simulink model "SpearheadSimulation"  (R2022a)
settings: Solver=ode4  StartTime=0.0  StopTime=250  RelTol=1e-3
values from neighbouring files (symbols this model uses):
  adb = importdata('datafiles/mga_v2_adb.dat')    [adbCoefficientModel.m]    (also in spearheadAnalysis.m = importdata('datafiles/adb_w_hat.txt'); spearheadControl.m = importdata('spearheadData/ConfigurationData/adb_w_hat.txt'); spearheadControl2.m = importdata('spearheadData/ConfigurationData/adb_w_hat.txt'); spearheadCruiseAnalysis.m = importdata('spearheadData/ConfigurationData/adb_w_hat.txt'))
  l_elevon = importdata('datafiles/le_w_hat.txt')    [spearheadAnalysis.m]    (also in spearheadControl.m = importdata('spearheadData/ConfigurationData/le_w_hat.txt'); spearheadControl2.m = importdata('spearheadData/ConfigurationData/le_w_hat.txt'); surfaceCoefficientModel.m = importdata('datafiles/l_elevon.dat'))
  r_elevon = importdata('datafiles/re_w_hat.txt')    [spearheadAnalysis.m]    (also in spearheadControl.m = importdata('spearheadData/ConfigurationData/re_w_hat.txt'); spearheadControl2.m = importdata('spearheadData/ConfigurationData/re_w_hat.txt'); surfaceCoefficientModel.m = importdata('datafiles/r_elevon.dat'))
  rudder = importdata('datafiles/rudder_w_hat.txt')    [spearheadAnalysis.m]    (also in spearheadControl.m = importdata('spearheadData/ConfigurationData/rudder_w_hat.txt; spearheadControl2.m = importdata('spearheadData/ConfigurationData/rudder_w_hat.txt; surfaceCoefficientModel.m = importdata('datafiles/rudder.dat'))
  T = pascal(max(dim,deg))    [makepolymat.m]    (also in spearheadAnalysis.m = 0.01; spearheadControl.m = 0.01; spearheadControl2.m = 0.01; spearheadVerticalAnalysis.m = 0.01)
libraries: slpidlib x19, simulink x5, vrlib x2, aerolibanim x1, aerolibanimutils x1
(part 2 of 2)

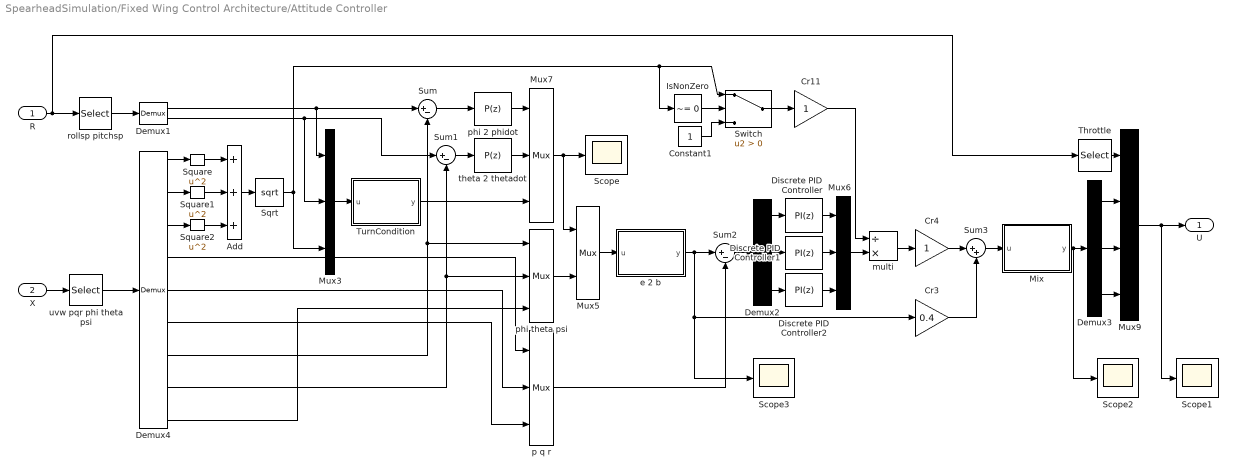
== system SpearheadSimulation/Fixed Wing Control Architecture/Attitude Controller ==
  R : Inport
  X : Inport  Port=2
  Add : Sum  Inputs=+++
  Constant1 : Constant
  Cr11 : Gain
  Cr3 : Gain  Gain=0.4
  Cr4 : Gain
  Demux1 : Demux  Outputs=2
  Demux2 : Demux  Outputs=3
  Demux3 : Demux  Outputs=3
  Demux4 : Demux  Outputs=9
  Discrete PID Controller : slpidlib/PID Controller  Controller=PI  Form=Parallel  TimeDomain=Discrete-time  UseExternalTs=off  SampleTime=-1  IntegratorMethod=Trapezoidal  FilterMethod=Trapezoidal  ControllerParametersSource=internal  P=5  I=0.5  UseKiTs=off  D=0  N=100  UseFilter=on  TunerSelectOption=Transfer Function Based (PID Tuner App)  InitialConditionSource=internal  InitialConditionForIntegrator=0  InitialConditionForFilter=0  DifferentiatorICPrevScaledInput=0  ExternalReset=none  TrackingMode=off  Kt=1  LimitOutput=off  SatLimitsSource=internal  UpperSaturationLimit=inf  LowerSaturationLimit=-inf  LinearizeAsGain=off  AntiWindupMode=none  Kb=1  POutMin=[]  POutMax=[]  IOutMin=[]  IOutMax=[]  DOutMin=[]  DOutMax=[]  NOutMin=[]  NOutMax=[]  SumOutMin=[]  SumOutMax=[]  SaturationOutMin=[]  SaturationOutMax=[]  PParamMin=[]  PParamMax=[]  IParamMin=[]  IParamMax=[]  DParamMin=[]  DParamMax=[]  NParamMin=[]  NParamMax=[]  KbParamMin=[]  KbParamMax=[]  KtParamMin=[]  KtParamMax=[]  KbOutMin=[]  KbOutMax=[]  KtOutMin=[]  KtOutMax=[]  IntegratorOutMin=[]  IntegratorOutMax=[]  FilterOutMin=[]  FilterOutMax=[]  SumI1OutMin=[]  SumI1OutMax=[]  SumI2OutMin=[]  SumI2OutMax=[]  SumI3OutMin=[]  SumI3OutMax=[]  SumI4OutMin=[]  SumI4OutMax=[]  SumDOutMin=[]  SumDOutMax=[]  DifferentiatorOutMin=[]  DifferentiatorOutMax=[]  FilterDiffOutCoefMin=[]  FilterDiffOutCoefMax=[]  ReciprocalOutMin=[]  ReciprocalOutMax=[]  SumDenOutMin=[]  SumDenOutMax=[]  SumNumOutMin=[]  SumNumOutMax=[]  DivideOutMin=[]  DivideOutMax=[]  UdiffTsProdOutMin=[]  UdiffTsProdOutMax=[]  NTsProdOutMin=[]  NTsProdOutMax=[]  UintegralTsProdOutMin=[]  UintegralTsProdOutMax=[]  UngainTsProdOutMin=[]  UngainTsProdOutMax=[]  IntegratorContinuousStateAttributes=''  IntegratorStateMustResolveToSignalObject=off  IntegratorRTWStateStorageClass=Auto  FilterContinuousStateAttributes=''  FilterStateMustResolveToSignalObject=off  FilterRTWStateStorageClass=Auto  ParallelPVariant=InternalParameters  IdealPVariant=Disabled  IVariant=InternalParameters  DVariant=Disabled  IntegratorVariant=Discrete  SatVariant=Disabled  AWVariant=Passthrough  PCopyVariant=Disabled  TRVariant=Disabled  FdbkBlocksVariant=Forward  IdealPFdbkVariant=Disabled  SatFdbkVariant=Disabled  DerivativeFilterVariant=Disabled  NVariant=Disabled  NCopyVariant=Disabled_SignalSpec  FilterICVariant=Disabled  IntegratorICVariant=InternalICs  ExternalResetVariant=Disabled  TRSumVariant=Passthrough  SumFdbkVariant=Disabled  SumVariant=Sum_PI  TsampFilterVariant=InternalTs  TsampNgainVariant=Passthrough  TsampIntegralVariant=Passthrough  ExternalSaturationOutDataTypeStr=Inherit: Same as second input  aMode=0
  Discrete PID Controller1 : slpidlib/PID Controller  Controller=PI  Form=Parallel  TimeDomain=Discrete-time  UseExternalTs=off  SampleTime=-1  IntegratorMethod=Trapezoidal  FilterMethod=Trapezoidal  ControllerParametersSource=internal  P=5  I=0.5  UseKiTs=off  D=0  N=100  UseFilter=on  TunerSelectOption=Transfer Function Based (PID Tuner App)  InitialConditionSource=internal  InitialConditionForIntegrator=0  InitialConditionForFilter=0  DifferentiatorICPrevScaledInput=0  ExternalReset=none  TrackingMode=off  Kt=1  LimitOutput=off  SatLimitsSource=internal  UpperSaturationLimit=inf  LowerSaturationLimit=-inf  LinearizeAsGain=off  AntiWindupMode=none  Kb=1  POutMin=[]  POutMax=[]  IOutMin=[]  IOutMax=[]  DOutMin=[]  DOutMax=[]  NOutMin=[]  NOutMax=[]  SumOutMin=[]  SumOutMax=[]  SaturationOutMin=[]  SaturationOutMax=[]  PParamMin=[]  PParamMax=[]  IParamMin=[]  IParamMax=[]  DParamMin=[]  DParamMax=[]  NParamMin=[]  NParamMax=[]  KbParamMin=[]  KbParamMax=[]  KtParamMin=[]  KtParamMax=[]  KbOutMin=[]  KbOutMax=[]  KtOutMin=[]  KtOutMax=[]  IntegratorOutMin=[]  IntegratorOutMax=[]  FilterOutMin=[]  FilterOutMax=[]  SumI1OutMin=[]  SumI1OutMax=[]  SumI2OutMin=[]  SumI2OutMax=[]  SumI3OutMin=[]  SumI3OutMax=[]  SumI4OutMin=[]  SumI4OutMax=[]  SumDOutMin=[]  SumDOutMax=[]  DifferentiatorOutMin=[]  DifferentiatorOutMax=[]  FilterDiffOutCoefMin=[]  FilterDiffOutCoefMax=[]  ReciprocalOutMin=[]  ReciprocalOutMax=[]  SumDenOutMin=[]  SumDenOutMax=[]  SumNumOutMin=[]  SumNumOutMax=[]  DivideOutMin=[]  DivideOutMax=[]  UdiffTsProdOutMin=[]  UdiffTsProdOutMax=[]  NTsProdOutMin=[]  NTsProdOutMax=[]  UintegralTsProdOutMin=[]  UintegralTsProdOutMax=[]  UngainTsProdOutMin=[]  UngainTsProdOutMax=[]  IntegratorContinuousStateAttributes=''  IntegratorStateMustResolveToSignalObject=off  IntegratorRTWStateStorageClass=Auto  FilterContinuousStateAttributes=''  FilterStateMustResolveToSignalObject=off  FilterRTWStateStorageClass=Auto  ParallelPVariant=InternalParameters  IdealPVariant=Disabled  IVariant=InternalParameters  DVariant=Disabled  IntegratorVariant=Discrete  SatVariant=Disabled  AWVariant=Passthrough  PCopyVariant=Disabled  TRVariant=Disabled  FdbkBlocksVariant=Forward  IdealPFdbkVariant=Disabled  SatFdbkVariant=Disabled  DerivativeFilterVariant=Disabled  NVariant=Disabled  NCopyVariant=Disabled_SignalSpec  FilterICVariant=Disabled  IntegratorICVariant=InternalICs  ExternalResetVariant=Disabled  TRSumVariant=Passthrough  SumFdbkVariant=Disabled  SumVariant=Sum_PI  TsampFilterVariant=InternalTs  TsampNgainVariant=Passthrough  TsampIntegralVariant=Passthrough  ExternalSaturationOutDataTypeStr=Inherit: Same as second input  aMode=0
  Discrete PID Controller2 : slpidlib/PID Controller  Controller=PI  Form=Parallel  TimeDomain=Discrete-time  UseExternalTs=off  SampleTime=-1  IntegratorMethod=Trapezoidal  FilterMethod=Trapezoidal  ControllerParametersSource=internal  P=5  I=0.5  UseKiTs=off  D=0  N=100  UseFilter=on  TunerSelectOption=Transfer Function Based (PID Tuner App)  InitialConditionSource=internal  InitialConditionForIntegrator=0  InitialConditionForFilter=0  DifferentiatorICPrevScaledInput=0  ExternalReset=none  TrackingMode=off  Kt=1  LimitOutput=off  SatLimitsSource=internal  UpperSaturationLimit=inf  LowerSaturationLimit=-inf  LinearizeAsGain=off  AntiWindupMode=none  Kb=1  POutMin=[]  POutMax=[]  IOutMin=[]  IOutMax=[]  DOutMin=[]  DOutMax=[]  NOutMin=[]  NOutMax=[]  SumOutMin=[]  SumOutMax=[]  SaturationOutMin=[]  SaturationOutMax=[]  PParamMin=[]  PParamMax=[]  IParamMin=[]  IParamMax=[]  DParamMin=[]  DParamMax=[]  NParamMin=[]  NParamMax=[]  KbParamMin=[]  KbParamMax=[]  KtParamMin=[]  KtParamMax=[]  KbOutMin=[]  KbOutMax=[]  KtOutMin=[]  KtOutMax=[]  IntegratorOutMin=[]  IntegratorOutMax=[]  FilterOutMin=[]  FilterOutMax=[]  SumI1OutMin=[]  SumI1OutMax=[]  SumI2OutMin=[]  SumI2OutMax=[]  SumI3OutMin=[]  SumI3OutMax=[]  SumI4OutMin=[]  SumI4OutMax=[]  SumDOutMin=[]  SumDOutMax=[]  DifferentiatorOutMin=[]  DifferentiatorOutMax=[]  FilterDiffOutCoefMin=[]  FilterDiffOutCoefMax=[]  ReciprocalOutMin=[]  ReciprocalOutMax=[]  SumDenOutMin=[]  SumDenOutMax=[]  SumNumOutMin=[]  SumNumOutMax=[]  DivideOutMin=[]  DivideOutMax=[]  UdiffTsProdOutMin=[]  UdiffTsProdOutMax=[]  NTsProdOutMin=[]  NTsProdOutMax=[]  UintegralTsProdOutMin=[]  UintegralTsProdOutMax=[]  UngainTsProdOutMin=[]  UngainTsProdOutMax=[]  IntegratorContinuousStateAttributes=''  IntegratorStateMustResolveToSignalObject=off  IntegratorRTWStateStorageClass=Auto  FilterContinuousStateAttributes=''  FilterStateMustResolveToSignalObject=off  FilterRTWStateStorageClass=Auto  ParallelPVariant=InternalParameters  IdealPVariant=Disabled  IVariant=InternalParameters  DVariant=Disabled  IntegratorVariant=Discrete  SatVariant=Disabled  AWVariant=Passthrough  PCopyVariant=Disabled  TRVariant=Disabled  FdbkBlocksVariant=Forward  IdealPFdbkVariant=Disabled  SatFdbkVariant=Disabled  DerivativeFilterVariant=Disabled  NVariant=Disabled  NCopyVariant=Disabled_SignalSpec  FilterICVariant=Disabled  IntegratorICVariant=InternalICs  ExternalResetVariant=Disabled  TRSumVariant=Passthrough  SumFdbkVariant=Disabled  SumVariant=Sum_PI  TsampFilterVariant=InternalTs  TsampNgainVariant=Passthrough  TsampIntegralVariant=Passthrough  ExternalSaturationOutDataTypeStr=Inherit: Same as second input  aMode=0
  IsNonZero : simulink/Logic and Bit Operations/Compare To Zero  relop=~=  OutDataTypeStr=boolean
  Mix : MATLAB Function  TreatAsAtomicUnit=on  SystemSampleTime=T
  Mux3 : Mux  Inputs=3
  Mux5 : Mux  Inputs=2
  Mux6 : Mux  Inputs=3
  Mux7 : Mux  Inputs=3
  Mux9 : Mux
  Scope{,1..3} (4 alike) : Scope
  Sqrt : Sqrt  OutputSignalType=real
  Square : Math  Operator=square
  Square1 : Math  Operator=square
  Square2 : Math  Operator=square
  Sum : Sum  Inputs=|+-
  Sum1 : Sum  Inputs=|+-
  Sum2 : Sum  Inputs=|+-
  Sum3 : Sum  Inputs=|++
  Switch : Switch  Criteria=u2 > Threshold  SaturateOnIntegerOverflow=off  InputSameDT=off
  Throttle : Selector  InputPortWidth=4  IndexOptions=Index vector (dialog)  Indices=[4]  OutputSizes=1
  TurnCondition : MATLAB Function  TreatAsAtomicUnit=on  SystemSampleTime=T
  e 2 b : MATLAB Function  TreatAsAtomicUnit=on  SystemSampleTime=T
  multi : Product  Inputs=/*
  p q r : Mux  Inputs=3
  phi 2 phidot : slpidlib/PID Controller  Controller=P  Form=Parallel  TimeDomain=Discrete-time  UseExternalTs=off  SampleTime=-1  IntegratorMethod=Trapezoidal  FilterMethod=Trapezoidal  ControllerParametersSource=internal  P=100  I=1  UseKiTs=off  D=0  N=100  UseFilter=on  TunerSelectOption=Transfer Function Based (PID Tuner App)  InitialConditionSource=internal  InitialConditionForIntegrator=0  InitialConditionForFilter=0  DifferentiatorICPrevScaledInput=0  ExternalReset=none  TrackingMode=off  Kt=1  LimitOutput=off  SatLimitsSource=internal  UpperSaturationLimit=inf  LowerSaturationLimit=-inf  LinearizeAsGain=off  AntiWindupMode=none  Kb=1  POutMin=[]  POutMax=[]  IOutMin=[]  IOutMax=[]  DOutMin=[]  DOutMax=[]  NOutMin=[]  NOutMax=[]  SumOutMin=[]  SumOutMax=[]  SaturationOutMin=[]  SaturationOutMax=[]  PParamMin=[]  PParamMax=[]  IParamMin=[]  IParamMax=[]  DParamMin=[]  DParamMax=[]  NParamMin=[]  NParamMax=[]  KbParamMin=[]  KbParamMax=[]  KtParamMin=[]  KtParamMax=[]  KbOutMin=[]  KbOutMax=[]  KtOutMin=[]  KtOutMax=[]  IntegratorOutMin=[]  IntegratorOutMax=[]  FilterOutMin=[]  FilterOutMax=[]  SumI1OutMin=[]  SumI1OutMax=[]  SumI2OutMin=[]  SumI2OutMax=[]  SumI3OutMin=[]  SumI3OutMax=[]  SumI4OutMin=[]  SumI4OutMax=[]  SumDOutMin=[]  SumDOutMax=[]  DifferentiatorOutMin=[]  DifferentiatorOutMax=[]  FilterDiffOutCoefMin=[]  FilterDiffOutCoefMax=[]  ReciprocalOutMin=[]  ReciprocalOutMax=[]  SumDenOutMin=[]  SumDenOutMax=[]  SumNumOutMin=[]  SumNumOutMax=[]  DivideOutMin=[]  DivideOutMax=[]  UdiffTsProdOutMin=[]  UdiffTsProdOutMax=[]  NTsProdOutMin=[]  NTsProdOutMax=[]  UintegralTsProdOutMin=[]  UintegralTsProdOutMax=[]  UngainTsProdOutMin=[]  UngainTsProdOutMax=[]  IntegratorContinuousStateAttributes=''  IntegratorStateMustResolveToSignalObject=off  IntegratorRTWStateStorageClass=Auto  FilterContinuousStateAttributes=''  FilterStateMustResolveToSignalObject=off  FilterRTWStateStorageClass=Auto  ParallelPVariant=InternalParameters  IdealPVariant=Disabled  IVariant=Disabled  DVariant=Disabled  IntegratorVariant=Disabled  SatVariant=Disabled  AWVariant=Disabled  PCopyVariant=Disabled  TRVariant=Disabled  FdbkBlocksVariant=Forward  IdealPFdbkVariant=Disabled  SatFdbkVariant=Disabled  DerivativeFilterVariant=Disabled  NVariant=Disabled  NCopyVariant=Disabled_SignalSpec  FilterICVariant=Disabled  IntegratorICVariant=Disabled  ExternalResetVariant=Disabled  TRSumVariant=Passthrough  SumFdbkVariant=Disabled  SumVariant=Passthrough_P  TsampFilterVariant=InternalTs  TsampNgainVariant=Passthrough  TsampIntegralVariant=Disabled_SignalSpec  ExternalSaturationOutDataTypeStr=Inherit: Same as second input  aMode=0
  phi theta psi : Mux  Inputs=3
  rollsp pitchsp : Selector  InputPortWidth=4  IndexOptions=Index vector (dialog)  Indices=[1,3]  OutputSizes=1
  theta 2 thetadot : slpidlib/PID Controller  Controller=P  Form=Parallel  TimeDomain=Discrete-time  UseExternalTs=off  SampleTime=-1  IntegratorMethod=Trapezoidal  FilterMethod=Trapezoidal  ControllerParametersSource=internal  P=100  I=1  UseKiTs=off  D=0  N=100  UseFilter=on  TunerSelectOption=Transfer Function Based (PID Tuner App)  InitialConditionSource=internal  InitialConditionForIntegrator=0  InitialConditionForFilter=0  DifferentiatorICPrevScaledInput=0  ExternalReset=none  TrackingMode=off  Kt=1  LimitOutput=off  SatLimitsSource=internal  UpperSaturationLimit=inf  LowerSaturationLimit=-inf  LinearizeAsGain=off  AntiWindupMode=none  Kb=1  POutMin=[]  POutMax=[]  IOutMin=[]  IOutMax=[]  DOutMin=[]  DOutMax=[]  NOutMin=[]  NOutMax=[]  SumOutMin=[]  SumOutMax=[]  SaturationOutMin=[]  SaturationOutMax=[]  PParamMin=[]  PParamMax=[]  IParamMin=[]  IParamMax=[]  DParamMin=[]  DParamMax=[]  NParamMin=[]  NParamMax=[]  KbParamMin=[]  KbParamMax=[]  KtParamMin=[]  KtParamMax=[]  KbOutMin=[]  KbOutMax=[]  KtOutMin=[]  KtOutMax=[]  IntegratorOutMin=[]  IntegratorOutMax=[]  FilterOutMin=[]  FilterOutMax=[]  SumI1OutMin=[]  SumI1OutMax=[]  SumI2OutMin=[]  SumI2OutMax=[]  SumI3OutMin=[]  SumI3OutMax=[]  SumI4OutMin=[]  SumI4OutMax=[]  SumDOutMin=[]  SumDOutMax=[]  DifferentiatorOutMin=[]  DifferentiatorOutMax=[]  FilterDiffOutCoefMin=[]  FilterDiffOutCoefMax=[]  ReciprocalOutMin=[]  ReciprocalOutMax=[]  SumDenOutMin=[]  SumDenOutMax=[]  SumNumOutMin=[]  SumNumOutMax=[]  DivideOutMin=[]  DivideOutMax=[]  UdiffTsProdOutMin=[]  UdiffTsProdOutMax=[]  NTsProdOutMin=[]  NTsProdOutMax=[]  UintegralTsProdOutMin=[]  UintegralTsProdOutMax=[]  UngainTsProdOutMin=[]  UngainTsProdOutMax=[]  IntegratorContinuousStateAttributes=''  IntegratorStateMustResolveToSignalObject=off  IntegratorRTWStateStorageClass=Auto  FilterContinuousStateAttributes=''  FilterStateMustResolveToSignalObject=off  FilterRTWStateStorageClass=Auto  ParallelPVariant=InternalParameters  IdealPVariant=Disabled  IVariant=Disabled  DVariant=Disabled  IntegratorVariant=Disabled  SatVariant=Disabled  AWVariant=Disabled  PCopyVariant=Disabled  TRVariant=Disabled  FdbkBlocksVariant=Forward  IdealPFdbkVariant=Disabled  SatFdbkVariant=Disabled  DerivativeFilterVariant=Disabled  NVariant=Disabled  NCopyVariant=Disabled_SignalSpec  FilterICVariant=Disabled  IntegratorICVariant=Disabled  ExternalResetVariant=Disabled  TRSumVariant=Passthrough  SumFdbkVariant=Disabled  SumVariant=Passthrough_P  TsampFilterVariant=InternalTs  TsampNgainVariant=Passthrough  TsampIntegralVariant=Disabled_SignalSpec  ExternalSaturationOutDataTypeStr=Inherit: Same as second input  aMode=0
  uvw pqr phi theta psi : Selector  InputPortWidth=20  IndexOptions=Index vector (dialog)  Indices=[1,2,3,4,5,6,10,11,12]  OutputSizes=1
  U : Outport
  wires:
  X/1 -> uvw pqr phi theta psi/1
  Sum1/1 -> theta 2 thetadot/1
  Sqrt/1 -> IsNonZero/1, Switch/1, Mux3/3
  Demux4/8 -> Sum1/2, phi theta psi/2
  Demux1/2 -> Sum1/1, Mux3/2
  Cr3/1 -> Sum3/2
  Mux7/1 -> Mux5/1, Scope/1
  Mux5/1 -> e 2 b/1(u)
  Cr4/1 -> Sum3/1
  rollsp pitchsp/1 -> Demux1/1
  R/1 -> rollsp pitchsp/1, Throttle/1
  Sum/1 -> phi 2 phidot/1
  Throttle/1 -> Mux9/1
  Demux4/5 -> p q r/2
  TurnCondition/1(y) -> Mux7/3
  multi/1 -> Cr4/1
  e 2 b/1(y) -> Sum2/1, Scope3/1, Cr3/1
  Demux3/1 -> Mux9/2
  phi theta psi/1 -> Mux5/2
  Mux9/1 -> Scope1/1, U/1
  Demux3/2 -> Mux9/3
  Demux4/2 -> Square1/1
  Demux1/1 -> Sum/1, Mux3/1
  Demux4/7 -> phi theta psi/1, Sum/2
  Mix/1(y) -> Scope2/1, Demux3/1
  phi 2 phidot/1 -> Mux7/1
  Mux3/1 -> TurnCondition/1(u)
  Square1/1 -> Add/2
  Sum2/1 -> Demux2/1
  Demux4/3 -> Square2/1
  Square/1 -> Add/1
  Square2/1 -> Add/3
  Add/1 -> Sqrt/1
  Demux4/4 -> p q r/1
  Sum3/1 -> Mix/1(u)
  Demux4/9 -> phi theta psi/3
  IsNonZero/1 -> Switch/2
  Demux3/3 -> Mux9/4
  Demux2/1 -> Discrete PID Controller/1
  Discrete PID Controller/1 -> Mux6/1
  Discrete PID Controller2/1 -> Mux6/3
  p q r/1 -> Sum2/2
  Switch/1 -> Cr11/1
  Demux2/3 -> Discrete PID Controller2/1
  Discrete PID Controller1/1 -> Mux6/2
  Mux6/1 -> multi/2
  Demux2/2 -> Discrete PID Controller1/1
  uvw pqr phi theta psi/1 -> Demux4/1
  Demux4/6 -> p q r/3
  Cr11/1 -> multi/1
  Demux4/1 -> Square/1
  Constant1/1 -> Switch/3
  theta 2 thetadot/1 -> Mux7/2

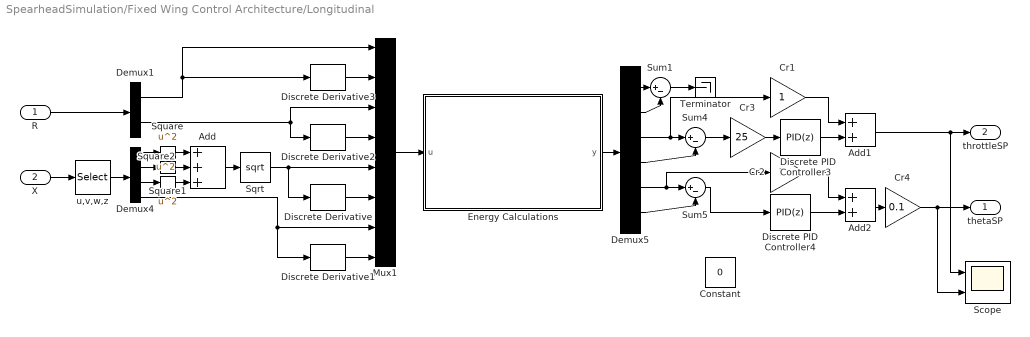
== system SpearheadSimulation/Fixed Wing Control Architecture/Longitudinal ==
  R : Inport
  X : Inport  Port=2
  Add : Sum  Inputs=+++
  Add1 : Sum
  Add2 : Sum
  Constant : Constant  Value=0
  Cr1 : Gain
  Cr2 : Gain
  Cr3 : Gain  Gain=25
  Cr4 : Gain  Gain=0.1
  Demux1 : Demux  Outputs=2
  Demux4 : Demux
  Demux5 : Demux  Outputs=6
  Discrete Derivative{,1..3} (4 alike) : simulink/Discrete/Discrete Derivative  gainval=1.0  ICPrevScaledInput=0.0  OutMin=[]  OutMax=[]  OutDataType=fixdt(1, 16)  OutScaling=2^-10  DoSatur=off
  Discrete PID Controller3 : slpidlib/PID Controller  Controller=PID  Form=Parallel  TimeDomain=Discrete-time  UseExternalTs=off  SampleTime=-1  IntegratorMethod=Trapezoidal  FilterMethod=Trapezoidal  ControllerParametersSource=internal  P=1  I=1/5  UseKiTs=off  D=1/25  N=100  UseFilter=on  TunerSelectOption=Transfer Function Based (PID Tuner App)  InitialConditionSource=internal  InitialConditionForIntegrator=0  InitialConditionForFilter=0  DifferentiatorICPrevScaledInput=0  ExternalReset=none  TrackingMode=off  Kt=1  LimitOutput=off  SatLimitsSource=internal  UpperSaturationLimit=inf  LowerSaturationLimit=-inf  LinearizeAsGain=off  AntiWindupMode=none  Kb=1  POutMin=[]  POutMax=[]  IOutMin=[]  IOutMax=[]  DOutMin=[]  DOutMax=[]  NOutMin=[]  NOutMax=[]  SumOutMin=[]  SumOutMax=[]  SaturationOutMin=[]  SaturationOutMax=[]  PParamMin=[]  PParamMax=[]  IParamMin=[]  IParamMax=[]  DParamMin=[]  DParamMax=[]  NParamMin=[]  NParamMax=[]  KbParamMin=[]  KbParamMax=[]  KtParamMin=[]  KtParamMax=[]  KbOutMin=[]  KbOutMax=[]  KtOutMin=[]  KtOutMax=[]  IntegratorOutMin=[]  IntegratorOutMax=[]  FilterOutMin=[]  FilterOutMax=[]  SumI1OutMin=[]  SumI1OutMax=[]  SumI2OutMin=[]  SumI2OutMax=[]  SumI3OutMin=[]  SumI3OutMax=[]  SumI4OutMin=[]  SumI4OutMax=[]  SumDOutMin=[]  SumDOutMax=[]  DifferentiatorOutMin=[]  DifferentiatorOutMax=[]  FilterDiffOutCoefMin=[]  FilterDiffOutCoefMax=[]  ReciprocalOutMin=[]  ReciprocalOutMax=[]  SumDenOutMin=[]  SumDenOutMax=[]  SumNumOutMin=[]  SumNumOutMax=[]  DivideOutMin=[]  DivideOutMax=[]  UdiffTsProdOutMin=[]  UdiffTsProdOutMax=[]  NTsProdOutMin=[]  NTsProdOutMax=[]  UintegralTsProdOutMin=[]  UintegralTsProdOutMax=[]  UngainTsProdOutMin=[]  UngainTsProdOutMax=[]  IntegratorContinuousStateAttributes=''  IntegratorStateMustResolveToSignalObject=off  IntegratorRTWStateStorageClass=Auto  FilterContinuousStateAttributes=''  FilterStateMustResolveToSignalObject=off  FilterRTWStateStorageClass=Auto  ParallelPVariant=InternalParameters  IdealPVariant=Disabled  IVariant=InternalParameters  DVariant=InternalParameters  IntegratorVariant=Discrete  SatVariant=Disabled  AWVariant=Passthrough  PCopyVariant=Disabled  TRVariant=Disabled  FdbkBlocksVariant=Forward  IdealPFdbkVariant=Disabled  SatFdbkVariant=Disabled  DerivativeFilterVariant=TrapezoidalFilter  NVariant=InternalParameters  NCopyVariant=InternalParameters  FilterICVariant=InternalICsFilter  IntegratorICVariant=InternalICs  ExternalResetVariant=Disabled  TRSumVariant=Passthrough  SumFdbkVariant=Disabled  SumVariant=Sum_PID  TsampFilterVariant=InternalTs  TsampNgainVariant=Passthrough  TsampIntegralVariant=Passthrough  ExternalSaturationOutDataTypeStr=Inherit: Same as second input  aMode=0
  Discrete PID Controller4 : slpidlib/PID Controller  Controller=PID  Form=Parallel  TimeDomain=Discrete-time  UseExternalTs=off  SampleTime=-1  IntegratorMethod=Trapezoidal  FilterMethod=Trapezoidal  ControllerParametersSource=internal  P=20  I=1  UseKiTs=off  D=10  N=100  UseFilter=on  TunerSelectOption=Transfer Function Based (PID Tuner App)  InitialConditionSource=internal  InitialConditionForIntegrator=0  InitialConditionForFilter=0  DifferentiatorICPrevScaledInput=0  ExternalReset=none  TrackingMode=off  Kt=1  LimitOutput=off  SatLimitsSource=internal  UpperSaturationLimit=inf  LowerSaturationLimit=-inf  LinearizeAsGain=off  AntiWindupMode=none  Kb=1  POutMin=[]  POutMax=[]  IOutMin=[]  IOutMax=[]  DOutMin=[]  DOutMax=[]  NOutMin=[]  NOutMax=[]  SumOutMin=[]  SumOutMax=[]  SaturationOutMin=[]  SaturationOutMax=[]  PParamMin=[]  PParamMax=[]  IParamMin=[]  IParamMax=[]  DParamMin=[]  DParamMax=[]  NParamMin=[]  NParamMax=[]  KbParamMin=[]  KbParamMax=[]  KtParamMin=[]  KtParamMax=[]  KbOutMin=[]  KbOutMax=[]  KtOutMin=[]  KtOutMax=[]  IntegratorOutMin=[]  IntegratorOutMax=[]  FilterOutMin=[]  FilterOutMax=[]  SumI1OutMin=[]  SumI1OutMax=[]  SumI2OutMin=[]  SumI2OutMax=[]  SumI3OutMin=[]  SumI3OutMax=[]  SumI4OutMin=[]  SumI4OutMax=[]  SumDOutMin=[]  SumDOutMax=[]  DifferentiatorOutMin=[]  DifferentiatorOutMax=[]  FilterDiffOutCoefMin=[]  FilterDiffOutCoefMax=[]  ReciprocalOutMin=[]  ReciprocalOutMax=[]  SumDenOutMin=[]  SumDenOutMax=[]  SumNumOutMin=[]  SumNumOutMax=[]  DivideOutMin=[]  DivideOutMax=[]  UdiffTsProdOutMin=[]  UdiffTsProdOutMax=[]  NTsProdOutMin=[]  NTsProdOutMax=[]  UintegralTsProdOutMin=[]  UintegralTsProdOutMax=[]  UngainTsProdOutMin=[]  UngainTsProdOutMax=[]  IntegratorContinuousStateAttributes=''  IntegratorStateMustResolveToSignalObject=off  IntegratorRTWStateStorageClass=Auto  FilterContinuousStateAttributes=''  FilterStateMustResolveToSignalObject=off  FilterRTWStateStorageClass=Auto  ParallelPVariant=InternalParameters  IdealPVariant=Disabled  IVariant=InternalParameters  DVariant=InternalParameters  IntegratorVariant=Discrete  SatVariant=Disabled  AWVariant=Passthrough  PCopyVariant=Disabled  TRVariant=Disabled  FdbkBlocksVariant=Forward  IdealPFdbkVariant=Disabled  SatFdbkVariant=Disabled  DerivativeFilterVariant=TrapezoidalFilter  NVariant=InternalParameters  NCopyVariant=InternalParameters  FilterICVariant=InternalICsFilter  IntegratorICVariant=InternalICs  ExternalResetVariant=Disabled  TRSumVariant=Passthrough  SumFdbkVariant=Disabled  SumVariant=Sum_PID  TsampFilterVariant=InternalTs  TsampNgainVariant=Passthrough  TsampIntegralVariant=Passthrough  ExternalSaturationOutDataTypeStr=Inherit: Same as second input  aMode=0
  Energy Calculations : MATLAB Function  TreatAsAtomicUnit=on  SystemSampleTime=T
  Mux1 : Mux  Inputs=8
  Scope : Scope  NumInputPorts=2
  Sqrt : Sqrt  OutputSignalType=real
  Square : Math  Operator=square
  Square1 : Math  Operator=square
  Square2 : Math  Operator=square
  Sum1 : Sum  Inputs=|+-
  Sum4 : Sum  Inputs=|+-
  Sum5 : Sum  Inputs=|+-
  Terminator : Terminator
  u,v,w,z : Selector  InputPortWidth=20  IndexOptions=Index vector (dialog)  Indices=[1,2,3,9]  OutputSizes=1
  thetaSP : Outport
  throttleSP : Outport  Port=2
  wires:
  X/1 -> u,v,w,z/1
  Demux4/2 -> Square1/1
  Square1/1 -> Add/2
  Demux4/3 -> Square2/1
  Square/1 -> Add/1
  Square2/1 -> Add/3
  Add/1 -> Sqrt/1
  u,v,w,z/1 -> Demux4/1
  Demux4/1 -> Square/1
  Mux1/1 -> Energy Calculations/1(u)
  Sqrt/1 -> Mux1/5, Discrete Derivative/1
  Demux4/4 -> Mux1/7, Discrete Derivative1/1
  R/1 -> Demux1/1
  Discrete Derivative1/1 -> Mux1/8
  Discrete Derivative/1 -> Mux1/6
  Demux1/2 -> Discrete Derivative2/1, Mux1/3
  Discrete Derivative2/1 -> Mux1/4
  Demux1/1 -> Discrete Derivative3/1, Mux1/1
  Discrete Derivative3/1 -> Mux1/2
  Energy Calculations/1(y) -> Demux5/1
  Demux5/1 -> Sum1/1
  Demux5/2 -> Sum1/2
  Demux5/3 -> Cr1/1, Sum4/1
  Demux5/4 -> Sum4/2
  Demux5/5 -> Cr2/1, Sum5/1
  Demux5/6 -> Sum5/2
  Discrete PID Controller3/1 -> Add1/2
  Cr1/1 -> Add1/1
  Add1/1 -> Scope/1, throttleSP/1
  Cr2/1 -> Add2/1
  Discrete PID Controller4/1 -> Add2/2
  Sum5/1 -> Discrete PID Controller4/1
  Cr3/1 -> Discrete PID Controller3/1
  Sum4/1 -> Cr3/1
  Sum1/1 -> Terminator/1
  Add2/1 -> Cr4/1
  Cr4/1 -> thetaSP/1, Scope/2

== matlab function SpearheadSimulation/SpearheadModel ==
  data: k input; dX output; X input; U input; adb input; l_elevon input; r_elevon input; rudder input
function dX  = spearheadModel(k,X,U,adb,l_elevon,r_elevon,rudder)
%% Xdot = f(X,U)

%% Mass of the VTOL Craft as Taken From CAD
M = 20;
g = 9.81;
rho = 1.225; % sea level air density

%% VTOL Dimensions
% CG at [0.6, 0, 0] m.
L1 = 1.65;
L2 = 1.425;
C = 0.32; % Wing Mean Cord Length
S = 2.24; % Wing Planform Area
eS = 0.28*0.58;% Elevon Planform Area chord x span
rS = 0.32*0.30;% Rudder Planform Area chord x span

%% Mass Moment of Inertia about the COM As Taken From CAD
Ixx = 5.061E+05;
Iyy = 5.061E+05;
Izz = 10.011E+05;

%% X = [u v w p q r x y z phi theta psi w1 w2 w3 w4 w5 dl dr drd]
% Linear and Angular Velocity in Fb (m/s and rads/s)
u = X(1);
v = X(2);
w = X(3);
p = X(4);
q = X(5);
r = X(6);
% Linear and Angular position in Fe (meters and rads)
x = X(7);
y = X(8);
z = X(9);
phi = X(10);
theta = X(11);
psi = X(12);
% Motor angular velocity (RPM)
w1 = X(13);
w2 = X(14);
w3 = X(15);
w4 = X(16);
w5 = X(17);
% Control Surface Defelection Angles(degrees)
dl = X(18);
dr = X(19);
drd = X(20);

%% U = [u1 u2 u3 u4 u5 u6 u7 u8] K = Motor Gain Mau = Time Constant Ku = Input Gain
K = [1.123*10^-6; 2.25*10^-6; 7.708*10^-7; 18.708*10^-7];
Mtau = [1/44.22; 1/44.22; 1/20];
Ku = [44.2205*8.18; 44.2205*7.02; 3.6];

F1 = K(1)*w1*w1;
F2 = K(1)*w2*w2;    
F3 = K(1)*w3*w3;
F4 = K(1)*w4*w4;

F5 = K(2)*w5*w5;

Tau1 = K(3)*w1*w1;
Tau2 = -K(3)*w2*w2;
Tau3 = -K(3)*w3*w3;
Tau4 = K(3)*w4*w4;

Tau5 = K(4)*w5*w5;

Fn = F1+F2+F3+F4;
Taun = Tau1+Tau2+Tau3+Tau4;

%% Wind Frame Variables: V = Airspeed alpha = AngleofAttack beta = AngleofSideslip
todeg = 180/pi;
V = sqrt(u*u + v*v + w*w);
alpha = atan2(w,u)*todeg;

if V == 0
  beta = 0;
else
  beta = asin(v/V)*todeg;
end

%% Aerodynamic Coefficients: ['CFX','CFY','CFZ','CMX','CMY','CMZ']
adb_C = adbCoefficients(alpha,beta,adb);
le_C = [1 dl dl^2 dl^3 dl^4 dl^5 dl^6 dl^7 dl^8]*l_elevon;
re_C = [1 dr dr^2 dr^3 dr^4 dr^5 dr^6 dr^7 dr^8]*r_elevon;
rudder_C = [1 drd drd^2 drd^3 drd^4 drd^5 drd^6 drd^7 drd^8]*rudder;

%% Forces: Thrust
FTx = F5;
FTy = 0;
FTz = -Fn;

%% Forces: Gravity
FGx = -g*sin(theta);
FGy = g*sin(phi)*cos(theta);
FGz = g*cos(phi)*cos(theta);

%% Forces: Aerodynamic [Drag,Sideforce,Lift]
FAx = 0.5 * rho * V*V * (S * adb_C(1) + eS * le_C(1) + eS * re_C(1) + rS * rudder_C(1));
FAy = 0.5 * rho * V*V * (S * adb_C(2) + eS * le_C(2) + eS * re_C(2) + rS * rudder_C(2));
FAz = 0.5 * rho * V*V * (S * adb_C(3) + eS * le_C(3) + eS * re_C(3) + rS * rudder_C(3));

%% Moments: Thrust
LT = L1*((F1 + F3) - (F2 + F4)) + Tau5;
MT = L2*((F1 + F2) - (F3 + F4));
NT = Taun;

%% Moments: Aerodynamic [Roll,Pitch,Yaw]
LA = 0.5 * rho * V*V * C * (S * adb_C(4) + eS * le_C(4) + eS * re_C(4) + rS * rudder_C(4));
MA = 0.5 * rho * V*V * C * (S * adb_C(5) + eS * le_C(5) + eS * re_C(5) + rS * rudder_C(5));
NA = 0.5 * rho * V*V * C * (S * adb_C(6) + eS * le_C(6) + eS * re_C(6) + rS * rudder_C(6));

%% 6-DOF Dynamics: dX = [udot vdot wdot pdot qdot rdot xdot ydot zdot phidot thetadot psidot]
dX1 = FGx + FAx/M + FTx/M - q*w + r*v;%# + g*sin(theta);
dX2 = FGy + FAy/M + FTy/M - r*u + p*w;
dX3 = FGz + FAz/M + FTz/M - p*v + q*u;%# - g*cos(theta);
dX4 = LA/Ixx + LT/Ixx - q*r*(Izz - Iyy)/Ixx;
dX5 = MA/Iyy + MT/Iyy - p*r*(Ixx - Izz)/Iyy;
dX6 = NA/Izz + NT/Izz - p*q*(Iyy - Ixx)/Izz;

dX7 = u*(cos(theta)*cos(psi)) + v*(sin(phi)*sin(theta)*cos(psi) - cos(phi)*sin(psi)) + w*(cos(phi)*sin(theta)*cos(psi) + sin(phi)*sin(psi));
dX8 = u*(cos(theta)*sin(psi)) + v*(sin(phi)*sin(theta)*sin(psi) + cos(phi)*cos(psi)) + w*(cos(phi)*sin(theta)*sin(psi) - sin(phi)*cos(psi));
dX9 = -u*(sin(theta)) + v*(sin(phi)*cos(theta)) + w*(cos(phi)*cos(theta));
dX10 = p + q*(sin(phi)*tan(theta)) + r*(cos(phi)*tan(theta));
dX11 = q*cos(phi) - r*sin(phi);
dX12 = q*(sin(phi)/cos(theta)) + r*(cos(phi)/cos(theta));

%% Motor Dynamics: dX = [w1dot w2dot w3dot w4dot w5dot], U = Pulse Width of the pwm signal 0-1000
dX13 = -(1/Mtau(1))*w1 + Ku(1)*U(1);
dX14 = -(1/Mtau(1))*w2 + Ku(1)*U(2);
dX15 = -(1/Mtau(1))*w3 + Ku(1)*U(3);
dX16 = -(1/Mtau(1))*w4 + Ku(1)*U(4);
dX17 = -(1/Mtau(2))*w5 + Ku(2)*U(5);

%% Servo Dynamics: dX = [w6dot w7dot w8dot], U = Pulse Width of the pwm signal 0-1000
dX18 = -(1/Mtau(3))*dl + Ku(3)*U(6);
dX19 = -(1/Mtau(3))*dr + Ku(3)*U(7);
dX20 = -(1/Mtau(3))*drd + Ku(3)*U(8);

dX = [dX1;dX2;dX3;dX4;dX5;dX6;dX7;dX8;dX9;dX10;dX11;dX12;dX13;dX14;dX15;dX16;dX17;dX18;dX19;dX20];
end

== matlab function SpearheadSimulation/Fixed Wing Control Architecture/Attitude Controller/e 2 b ==
  data: u input; y output
function y = etb(u)
y = [1,sin(u(4))*tan(u(5)),cos(u(4))*tan(u(5));
     0,            cos(u(4)),           -sin(u(4));
     0,sin(u(4))/cos(u(5)),cos(u(4))/cos(u(5))]\u([1,2,3]);

== matlab function SpearheadSimulation/Fixed Wing Control Architecture/Attitude Controller/TurnCondition ==
  data: u input; y output
function y = TurnCondition(u)

if u(3) == 0
    y = 0;
else
    y = (9.81/u(3)) * tan(u(1)) * cos(u(2));
end

== matlab function SpearheadSimulation/Fixed Wing Control Architecture/Attitude Controller/Mix ==
  data: u input; y output
function y = Mix(u)
y = [0.5,0.5,0;
     -0.5,0.5,0;
     0,0,1]*u;

== matlab function SpearheadSimulation/Fixed Wing Control Architecture/Longitudinal/Energy Calculations ==
  data: u input; y output
function y = Energy(u)
M = 20;
g = 9.81;

hsp = u(3);
hdotsp = u(4);
h = u(7);
hdot = u(8);
Vsp = u(1);
Vdot = u(2);
V = u(5);
Vdotsp = u(6);

Et = 0.5 * M * V^2 + M * g * h;
Etdot = M * V * Vdot + M * g * hdot;
if V == 0 
    Edot = 0;
    gamma  = 0;
else
    Edot = Etdot/(M * g * V);
    gamma = asin(abs(hdot/V));
end
Bdot = gamma - Vdot/g;

Etsp = 0.5 * M * Vsp^2 + M * g * hsp;
Etdotsp = M * Vsp * Vdotsp + M * g * hdotsp;
if Vsp == 0
    Edotsp = 0;
    gammasp  = 0;
else
    Edotsp = Etdotsp/(M * g * V);
    gammasp = asin(abs(hdotsp/Vsp));
end        
Bdotsp = gammasp - Vdotsp/g;

y = [Etsp,Et,Edotsp,Edot,Bdotsp,Bdot];
end

== matlab function SpearheadSimulation/Rotor Wing Control Architecture/Acceleration to Attitiude ==
  data: u input; y output
function y = ata(u)

collcmd =  sqrt((u(1)^2)*(u(2)^2)*(u(3)^2));

if collcmd == 0
    I = [0;0;0];
else
    I = u([1;2;3])/collcmd;
end

K = [cos(u(4)),sin(u(4)),0;
     -sin(u(4)),cos(u(4)),0;
     0,         0,       1]*I;

if collcmd == 0
    thetacmd = 0;
else
    thetacmd = atan(K(1)/K(3));
end

L = [cos(thetacmd),0,-sin(thetacmd);
        0,         1,       0;
     sin(thetacmd),0,cos(thetacmd)]*K;

if collcmd == 0
    phicmd = 0;
else
    phicmd = atan2(-L(2),L(3));
end

y = [phicmd,thetacmd,u(4),u(3)];

end

== matlab function SpearheadSimulation/Rotor Wing Control Architecture/Mix1 ==
  data: u input; y output
function y = Mix(u)
M = 20;
L1 = 1.65;
L2 = 1.425;
Ixx = 5.061E+05;
Iyy = 5.061E+05;
Izz = 10.011E+05;
K = 1.123*10^-6;
K2 = 7.708*10^-7;
Ku = 44.2205*8.18;

%{
Usqr = [L1*K/Ixx, -L1*K/Ixx, L1*K/Ixx, -L1*K/Ixx;
        L2*K/Iyy, L2*K/Iyy, -L2*K/Iyy, -L2*K/Iyy;
        K2/Izz,    -K2/Izz,   -K2/Izz,    K2/Izz;
        -K/M,      -K/M,      -K/M,      -K/M]\u;
%}

Usqr = [(u(1) + u(2) + u(3) - u(4));
        (-u(1) + u(2) - u(3) - u(4));
        (u(1) - u(2) - u(3) - u(4));
        (-u(1) - u(2) + u(3) - u(4))];

%{
Usqr = [((L1/Ixx)*K*Ku*u(1) + (L2/Iyy)*K*Ku*u(2) + (1/Izz)*K2*Ku*u(3) - M*Ku*K*u(4));
        (-(L1/Ixx)*K*Ku*u(1) + (L2/Iyy)*K*Ku*u(2) - (1/Izz)*K2*Ku*u(3) - M*Ku*K*u(4));
        ((L1/Ixx)*K*Ku*u(1) - (L2/Iyy)*K*Ku*u(2) - (1/Izz)*K2*Ku*u(3) - M*Ku*K*u(4));
        (-(L1/Ixx)*K*Ku*u(1) - (L2/Iyy)*K*Ku*u(2) + (1/Izz)*K2*Ku*u(3) - M*Ku*K*u(4))];
%}
%y = sqrt(abs(Usqr))/Ku;

y = Usqr;
